simulink library "casper_library"  (Simulink 6.2)
PostLoadFcn:
  | % Stub definitions for mask variables
  | delay_depth=16;
  | n_bits=8;
  | bin_pt=7;
values from neighbouring files (symbols this model uses):
  add_latency = get_var('add_latency', 'defaults', defaults, varargin{:})    [biplex_core_init.m]    (also in butterfly_direct_init.m; dec_fir_init.m = get_var('add_latency','defaults', defaults, varargin{:}); fft_biplex_real_4x_init.m; fft_direct_init.m)
  BitWidth = get_var('BitWidth', 'defaults', defaults, varargin{:})    [biplex_core_init.m]    (also in butterfly_direct_init.m; fft_biplex_init.m; fft_biplex_real_2x_init.m; fft_biplex_real_4x_init.m)
  blockCountBits = ceil(log2(numBlocks))    [address_gen_vacc_v2_mask.m]
  blockRowBits = 0    [address_gen_vacc_v2_mask.m]
  mult_latency = get_var('mult_latency', 'defaults', defaults, varargin{:})    [biplex_core_init.m]    (also in butterfly_direct_init.m; dec_fir_init.m = get_var('mult_latency','defaults', defaults, varargin{:}); fft_biplex_real_4x_init.m; fft_direct_init.m)
  n_inputs = get_var('n_inputs', 'defaults', defaults, varargin{:})    [adder_tree_init.m]    (also in barrel_switcher_init.m; dec_fir_init.m = get_var('n_inputs','defaults', defaults, varargin{:}); fft_init.m; fft_unscrambler_init.m)
undefined symbols (not defined in the file or in its folder): acc_len, ant_bits, bit_growth, bit_rev, BitWidthIn, cmult_4bit_br, cmult_4bit_em, cmult_4bit_sl, CoeffBitWidth, DelayLen, n_ants, n_bits_out, pfb_coeff_gen_calc, PFBSize
libraries: xbsIndex_r3 x2630, casper_library x215, xps_library x24, fft_library x4
(part 5 of 21)

== system casper_library/Misc/adder_tree ==
  sync : Inport  Port=1  LatchInput=off
  din1 : Inport  Port=2  LatchInput=off
  din2 : Inport  Port=3  LatchInput=off
  addr1 : xbsIndex_r3/AddSub  mode=Addition  precision=Full  arith_type=Unsigned  n_bits=8  bin_pt=2  quantization=Truncate  overflow=Wrap  latency=1  explicit_period=off  period=1  use_carryin=off  use_carryout=off  en=off  dbl_ovrd=off  show_param=off  use_core=on  pipeline=on  use_rpm=on  gen_core=off
      settings: xl_area=[0, 0, 0, 0, 0, 0, 0]
  sync_delay : xbsIndex_r3/Delay  latency=1  reg_retiming=off  explicit_period=off  period=1  en=off  accept_only_valid=off  init_zero=on  dbl_ovrd=off  show_param=off
      settings: xl_area=[0, 0, 0, 0, 0, 0, 0]
  sync_out : Outport
  dout : Outport  Port=2
  wires:
  sync/1 -> sync_delay/1
  sync_delay/1 -> sync_out/1
  din1/1 -> addr1/1
  din2/1 -> addr1/2
  addr1/1 -> dout/1

== system casper_library/Misc/bit_reverse ==
  in : Inport  Port=1  LatchInput=off
  out : Outport
  wires:
  in/1 -> out/1

== system casper_library/Misc/c_to_ri ==
  c : Inport  Port=1  LatchInput=off
  force_im : xbsIndex_r3/Reinterpret  force_arith_type=on  arith_type="Signed  (2's comp)"  force_bin_pt=on  bin_pt=bin_pt  force_valid=on
  force_re : xbsIndex_r3/Reinterpret  force_arith_type=on  arith_type="Signed  (2's comp)"  force_bin_pt=on  bin_pt=bin_pt  force_valid=on
  slice_im : xbsIndex_r3/Slice  mode=Lower Bit Location + Width  nbits=n_bits  bit1=0  base1=MSB of Input  bit0=0  base0=LSB of Input  boolean_output=off  explicit_period=off  period=1  dbl_ovrd=off
  slice_re : xbsIndex_r3/Slice  mode=Upper Bit Location + Width  nbits=n_bits  bit1=0  base1=MSB of Input  bit0=0  base0=LSB of Input  boolean_output=off  explicit_period=off  period=1  dbl_ovrd=off
  re : Outport
  im : Outport  Port=2
  wires:
  slice_re/1 -> force_re/1
  slice_im/1 -> force_im/1
  force_re/1 -> re/1
  force_im/1 -> im/1
  c/1 -> slice_re/1, slice_im/1

== system casper_library/Misc/complex_addsub ==
  a : Inport  Port=1  LatchInput=off
  b : Inport  Port=2  LatchInput=off
  AddSub : xbsIndex_r3/AddSub  mode=Addition  precision=Full  arith_type=Unsigned  n_bits=8  bin_pt=2  quantization=Truncate  overflow=Wrap  latency=add_latency  explicit_period=off  period=1  use_carryin=off  use_carryout=off  en=off  dbl_ovrd=off  show_param=off  use_core=on  pipeline=off  use_rpm=on  gen_core=off
      settings: xl_area=[0, 0, 0, 0, 0, 0, 0]
  AddSub1 : xbsIndex_r3/AddSub  mode=Subtraction  precision=Full  arith_type=Unsigned  n_bits=8  bin_pt=2  quantization=Truncate  overflow=Wrap  latency=add_latency  explicit_period=off  period=1  use_carryin=off  use_carryout=off  en=off  dbl_ovrd=off  show_param=off  use_core=on  pipeline=off  use_rpm=on  gen_core=off
      settings: xl_area=[0, 0, 0, 0, 0, 0, 0]
  AddSub2 : xbsIndex_r3/AddSub  mode=Subtraction  precision=Full  arith_type=Unsigned  n_bits=8  bin_pt=2  quantization=Truncate  overflow=Wrap  latency=add_latency  explicit_period=off  period=1  use_carryin=off  use_carryout=off  en=off  dbl_ovrd=off  show_param=off  use_core=on  pipeline=off  use_rpm=on  gen_core=off
      settings: xl_area=[0, 0, 0, 0, 0, 0, 0]
  AddSub3 : xbsIndex_r3/AddSub  mode=Addition  precision=Full  arith_type=Unsigned  n_bits=8  bin_pt=2  quantization=Truncate  overflow=Wrap  latency=add_latency  explicit_period=off  period=1  use_carryin=off  use_carryout=off  en=off  dbl_ovrd=off  show_param=off  use_core=on  pipeline=off  use_rpm=on  gen_core=off
      settings: xl_area=[0, 0, 0, 0, 0, 0, 0]
  Convert{,1..3} (4 alike) : xbsIndex_r3/Convert  arith_type="Signed  (2's comp)"  n_bits=BitWidth  bin_pt=BitWidth - 1  quantization="Round  (unbiased: Even Values)"  overflow=Wrap  latency=add_latency  explicit_period=off  period=1  dbl_ovrd=off  show_param=off  inserted_by_tool=off  pipeline=off
      settings: xl_area=[0, 0, 0, 0, 0, 0, 0]
  Shift{,1..3} (4 alike) : xbsIndex_r3/Shift  shift_dir=Right  shift_bits=1  precision=Full  arith_type="Signed  (2's comp)"  n_bits=8  bin_pt=2  quantization=Truncate  overflow=Wrap  latency=0  explicit_period=off  period=1  en=off  dbl_ovrd=off  show_param=off
      settings: xl_area=[0, 0, 0, 0, 0, 0, 0]
  c_to_ri : casper_library/Misc/c_to_ri  n_bits=BitWidth  bin_pt=BitWidth-1
      settings: AttributesFormatString=18_17 r/i
  c_to_ri1 : casper_library/Misc/c_to_ri  n_bits=BitWidth  bin_pt=BitWidth-1
      settings: AttributesFormatString=18_17 r/i
  ri_to_c : casper_library/Misc/ri_to_c
  ri_to_c1 : casper_library/Misc/ri_to_c
  a+b : Outport
  a-b : Outport  Port=2
  wires:
  Shift3/1 -> Convert3/1
  Shift2/1 -> Convert2/1
  Shift1/1 -> Convert1/1
  Shift/1 -> Convert/1
  b/1 -> c_to_ri1/1
  ri_to_c1/1 -> a-b/1
  ri_to_c/1 -> a+b/1
  a/1 -> c_to_ri/1
  Convert2/1 -> ri_to_c/2
  Convert/1 -> ri_to_c/1
  c_to_ri1/2 -> AddSub3/2, AddSub2/2
  c_to_ri1/1 -> AddSub/2, AddSub1/1
  c_to_ri/2 -> AddSub3/1, AddSub2/1
  c_to_ri/1 -> AddSub/1, AddSub1/2
  AddSub3/1 -> Shift3/1
  AddSub2/1 -> Shift2/1
  AddSub1/1 -> Shift1/1
  AddSub/1 -> Shift/1
  Convert1/1 -> ri_to_c1/2
  Convert3/1 -> ri_to_c1/1

== system casper_library/Misc/cram ==
  In1 : Inport  Port=1  LatchInput=off
  In2 : Inport  Port=2  LatchInput=off
  In3 : Inport  Port=3  LatchInput=off
  In4 : Inport  Port=4  LatchInput=off
  Concat : S-Function  AncestorBlock=xbsIndex_r3/Concat  FunctionName=xlconcat  Parameters=sfcn_mwsv__  mask(Xilinx Bus Concatenator){num_inputs=4, explicit_period=off, period=1, dbl_ovrd=off}
      mask prompts: num_inputs "Number of Inputs"; explicit_period "Use Explicit Sample Period"; period "Sample Period  (use -1 to inherit first known input period)"; dbl_ovrd "Override with Doubles"
      mask help: Concatenates two or more inputs. Inputs must be unsigned with binary point at zero.
      mask init:
      | [designRoot, family, part, speed, package, simulinkPeriod, sysclkPeriod, dbl_ovrd, trimVbit] = xlSysgenSettings(gcb,1,1);
      | [bg,fg] = xlcmap('XBlock',dbl_ovrd);
      | iPos = get_param(gcb,'Position');
      | iWidth=iPos(3)-iPos(1); iHeight=iPos(4)-iPos(2);
      | iCx=iWidth/2;
      | iCy=iHeight/2;
      | [logoX, logoY] = xlogo(iPos);
      | 
      | 
      | 
      | 
      | % one time added for param list
      | numInputs = num_inputs + 1;
      | precision0 = 1;
      | latency = 0;
      | dblOvrd = dbl_ovrd;
      | explicitClk = explicit_period;
      | 
      | 
      | % just pass everything to s-function
      | sfcn_mwsv__ = get_param(gcb, 'MaskWSVariables');
      mask Help: eval('xlWeb(xlhtmldoclink(''Concat''))');
      mask StyleString: popup(2|3|4|5|6|7|8|9|10|11|12|13|14|15|16),checkbox,edit,checkbox
      mask CallbackString: |xlMagicCallback||
      mask Display:
      | patch([0 iWidth iWidth 0],[0 0 iHeight iHeight] , bg);
      | patch(logoX,logoY, fg);
      | port_label('input',1,'hi');
      | port_label('input',num_inputs+1,'lo');
      | port_label('output',1,'cat');
      | ;plot([0 0 iWidth iWidth 0], [0 iHeight iHeight 0 0]);
  Reinterp{1..4} (4 alike) : xbsIndex_r3/Reinterpret  force_arith_type=on  arith_type=Unsigned  force_bin_pt=on  bin_pt=0  force_valid=on
  Out : Outport
  wires:
  Concat/1 -> Out/1
  In1/1 -> Reinterp1/1
  Reinterp1/1 -> Concat/1
  In2/1 -> Reinterp2/1
  Reinterp2/1 -> Concat/2
  In3/1 -> Reinterp3/1
  Reinterp3/1 -> Concat/3
  In4/1 -> Reinterp4/1
  Reinterp4/1 -> Concat/4

== system casper_library/Misc/edge ==
  in : Inport  Port=1  LatchInput=off
  Delay4 : xbsIndex_r3/Delay  latency=1  reg_retiming=off  explicit_period=off  period=1  en=off  accept_only_valid=off  init_zero=on  dbl_ovrd=off  show_param=off
      settings: xl_area=[0, 0, 0, 0, 0, 0, 0]
  Logical3 : xbsIndex_r3/Logical  logical_function=XOR  inputs=2  precision=Full  arith_type=Unsigned  n_bits=8  bin_pt=2  align_bp=on  latency=0  explicit_period=off  period=1  en=off  dbl_ovrd=off  show_param=off
      settings: xl_area=[0, 0, 0, 0, 0, 0, 0]
  out : Outport
  wires:
  Logical3/1 -> out/1
  Delay4/1 -> Logical3/1
  in/1 -> Delay4/1, Logical3/2

== system casper_library/Misc/freeze_cntr ==
  en : Inport  Port=1  LatchInput=off
  rst : Inport  Port=2  LatchInput=off
  Counter3 : xbsIndex_r3/Counter  cnt_type=Free Running  n_bits=CounterBits + 1  bin_pt=0  arith_type=Unsigned  start_count=0  cnt_to=1023  cnt_by_val=1  operation=Up  explicit_period=on  period=1  load_pin=off  rst=on  en=on  dbl_ovrd=off  show_param=off  use_rpm=on  gen_core=off
      settings: xl_area=[0, 0, 0, 0, 0, 0, 0]
  Inverter : xbsIndex_r3/Inverter  latency=0  explicit_period=off  period=1  en=off  dbl_ovrd=off  show_param=off
      settings: xl_area=[0, 0, 0, 0, 0, 0, 0]
  Inverter1 : xbsIndex_r3/Inverter  latency=0  explicit_period=off  period=1  en=off  dbl_ovrd=off  show_param=off
      settings: xl_area=[0, 0, 0, 0, 0, 0, 0]
  Logical1 : xbsIndex_r3/Logical  logical_function=AND  inputs=2  precision=Full  arith_type=Unsigned  n_bits=8  bin_pt=2  align_bp=on  latency=0  explicit_period=off  period=1  en=off  dbl_ovrd=off  show_param=off
      settings: xl_area=[0, 0, 0, 0, 0, 0, 0]
  Logical5 : xbsIndex_r3/Logical  logical_function=AND  inputs=2  precision=Full  arith_type=Unsigned  n_bits=8  bin_pt=2  align_bp=on  latency=0  explicit_period=off  period=1  en=off  dbl_ovrd=off  show_param=off
      settings: xl_area=[0, 0, 0, 0, 0, 0, 0]
  enable : xbsIndex_r3/Slice  mode=Lower Bit Location + Width  nbits=CounterBits  bit1=0  base1=LSB of Input  bit0=0  base0=LSB of Input  boolean_output=off  explicit_period=off  period=1  dbl_ovrd=off
  enable1 : xbsIndex_r3/Slice  mode=Upper Bit Location + Width  nbits=1  bit1=0  base1=MSB of Input  bit0=0  base0=LSB of Input  boolean_output=on  explicit_period=off  period=1  dbl_ovrd=off
  addr : Outport
  we : Outport  Port=2
  done : Outport  Port=3
  wires:
  Logical1/1 -> we/1
  Inverter/1 -> Logical1/1
  Counter3/1 -> enable1/1, enable/1
  enable1/1 -> Inverter1/1, done/1
  en/1 -> Logical5/1
  Logical5/1 -> Logical1/2, Counter3/2
  rst/1 -> Inverter/1, Counter3/1
  enable/1 -> addr/1
  Inverter1/1 -> Logical5/2

== system casper_library/Misc/negedge ==
  In : Inport  Port=1  LatchInput=off
  Delay : xbsIndex_r3/Delay  latency=1  reg_retiming=off  explicit_period=off  period=1  en=off  accept_only_valid=off  init_zero=on  dbl_ovrd=off  show_param=off
      settings: xl_area=[0, 0, 0, 0, 0, 0, 0]
  Inverter : xbsIndex_r3/Inverter  latency=0  explicit_period=off  period=1  en=off  dbl_ovrd=off  show_param=off
      settings: xl_area=[0, 0, 0, 0, 0, 0, 0]
  Logical : xbsIndex_r3/Logical  logical_function=AND  inputs=2  precision=Full  arith_type=Unsigned  n_bits=8  bin_pt=2  align_bp=on  latency=0  explicit_period=off  period=1  en=off  dbl_ovrd=off  show_param=off
      settings: xl_area=[0, 0, 0, 0, 0, 0, 0]
  Out : Outport
  wires:
  Delay/1 -> Logical/1
  In/1 -> Delay/1, Inverter/1
  Logical/1 -> Out/1
  Inverter/1 -> Logical/2

== system casper_library/Misc/posedge ==
  In : Inport  Port=1  LatchInput=off
  Delay : xbsIndex_r3/Delay  latency=1  reg_retiming=off  explicit_period=off  period=1  en=off  accept_only_valid=off  init_zero=on  dbl_ovrd=off  show_param=off
      settings: xl_area=[0, 0, 0, 0, 0, 0, 0]
  Inverter : xbsIndex_r3/Inverter  latency=0  explicit_period=off  period=1  en=off  dbl_ovrd=off  show_param=off
      settings: xl_area=[0, 0, 0, 0, 0, 0, 0]
  Logical : xbsIndex_r3/Logical  logical_function=AND  inputs=2  precision=Full  arith_type=Unsigned  n_bits=8  bin_pt=2  align_bp=on  latency=0  explicit_period=off  period=1  en=off  dbl_ovrd=off  show_param=off
      settings: xl_area=[0, 0, 0, 0, 0, 0, 0]
  Out : Outport
  wires:
  Logical/1 -> Out/1
  In/1 -> Logical/2, Delay/1
  Inverter/1 -> Logical/1
  Delay/1 -> Inverter/1

== system casper_library/Misc/power ==
  c : Inport  Port=1  LatchInput=off
  c_to_ri : casper_library/Misc/c_to_ri  n_bits=BitWidth  bin_pt=BitWidth-1
      settings: AttributesFormatString=18_17 r/i
  imag_square : xbsIndex_r3/Mult  precision=Full  arith_type="Signed  (2's comp)"  n_bits=8  bin_pt=2  quantization=Truncate  overflow=Wrap  latency=3  explicit_period=off  period=1  en=off  dbl_ovrd=off  show_param=on  mult_type=Parallel  oversample=2  use_embedded=on  pipeline=on  use_rpm=on  placement_style=Rectangular Shape  gen_core=off
      settings: xl_area=[0, 0, 0, 0, 0, 0, 0]
  power_adder : xbsIndex_r3/AddSub  mode=Addition  precision=User Defined  arith_type=Unsigned  n_bits=BitWidth * 2  bin_pt=BitWidth * 2 - 1  quantization=Truncate  overflow=Wrap  latency=2  explicit_period=off  period=1  use_carryin=off  use_carryout=off  en=off  dbl_ovrd=off  show_param=off  use_core=on  pipeline=off  use_rpm=on  gen_core=off
      settings: xl_area=[0, 0, 0, 0, 0, 0, 0]
  real_square : xbsIndex_r3/Mult  precision=Full  arith_type="Signed  (2's comp)"  n_bits=8  bin_pt=2  quantization=Truncate  overflow=Wrap  latency=3  explicit_period=off  period=1  en=off  dbl_ovrd=off  show_param=on  mult_type=Parallel  oversample=2  use_embedded=on  pipeline=on  use_rpm=on  placement_style=Rectangular Shape  gen_core=off
      settings: xl_area=[0, 0, 0, 0, 0, 0, 0]
  power : Outport
  wires:
  c_to_ri/2 -> imag_square/1, imag_square/2
  c_to_ri/1 -> real_square/2, real_square/1
  c/1 -> c_to_ri/1
  real_square/1 -> power_adder/1
  imag_square/1 -> power_adder/2
  power_adder/1 -> power/1

== system casper_library/Misc/pulse_ext ==
  in : Inport  Port=1  LatchInput=off
  Constant5 : xbsIndex_r3/Constant  const=pulse_len  equ=P=C  arith_type=Unsigned  n_bits=bits  bin_pt=0  opselect=C  inp2=PCIN>>17  opr=+  inp1=P  carry=CIN  iostate=0  explicit_period=off  period=1  dbl_ovrd=off
  Counter3 : xbsIndex_r3/Counter  cnt_type=Free Running  n_bits=bits  bin_pt=0  arith_type=Unsigned  start_count=0  cnt_to=1023  cnt_by_val=1  operation=Up  explicit_period=on  period=1  load_pin=off  rst=on  en=on  dbl_ovrd=off  show_param=off  use_rpm=on  gen_core=off
      settings: xl_area=[0, 0, 0, 0, 0, 0, 0]
  Relational5 : xbsIndex_r3/Relational  mode=a!=b  latency=0  explicit_period=off  period=1  en=off  dbl_ovrd=off  show_param=off
      settings: xl_area=[0, 0, 0, 0, 0, 0, 0]
  posedge : Subsystem  Tag=Rising Edge Detector
  out : Outport
  wires:
  Counter3/1 -> Relational5/1
  Constant5/1 -> Relational5/2
  Relational5/1 -> Counter3/2, out/1
  in/1 -> posedge/1(In)
  posedge/1(Out) -> Counter3/1

== system casper_library/Misc/ri_to_c ==
  re : Inport  Port=1  LatchInput=off
  im : Inport  Port=2  LatchInput=off
  concat : xbsIndex_r3/Concat  num_inputs=2  explicit_period=off  period=1  dbl_ovrd=off
  force_im : xbsIndex_r3/Reinterpret  force_arith_type=on  arith_type=Unsigned  force_bin_pt=on  bin_pt=0  force_valid=on
  force_re : xbsIndex_r3/Reinterpret  force_arith_type=on  arith_type=Unsigned  force_bin_pt=on  bin_pt=0  force_valid=on
  c : Outport
  wires:
  force_re/1 -> concat/1
  force_im/1 -> concat/2
  re/1 -> force_re/1
  concat/1 -> c/1
  im/1 -> force_im/1

== system casper_library/Misc/stopwatch ==
  start : Inport  Port=1  LatchInput=off
  stop : Inport  Port=2  LatchInput=off
  reset : Inport  Port=3  LatchInput=off
  Constant1 : xbsIndex_r3/Constant  const=1  equ=P=C  arith_type=Boolean  n_bits=1  bin_pt=0  opselect=C  inp2=PCIN>>17  opr=+  inp1=P  carry=CIN  iostate=0  explicit_period=on  period=1  dbl_ovrd=off
  Constant8 : xbsIndex_r3/Constant  const=1  equ=P=C  arith_type=Boolean  n_bits=1  bin_pt=0  opselect=C  inp2=PCIN>>17  opr=+  inp1=P  carry=CIN  iostate=0  explicit_period=on  period=1  dbl_ovrd=off
  Counter1 : xbsIndex_r3/Counter  cnt_type=Free Running  n_bits=32  bin_pt=0  arith_type=Unsigned  start_count=0  cnt_to=Inf  cnt_by_val=1  operation=Up  explicit_period=off  period=1  load_pin=off  rst=on  en=on  dbl_ovrd=off  show_param=off  use_rpm=on  gen_core=off
      settings: xl_area=[0, 0, 0, 0, 0, 0, 0]
  Logical : xbsIndex_r3/Logical  logical_function=AND  inputs=2  precision=Full  arith_type=Unsigned  n_bits=8  bin_pt=2  align_bp=on  latency=0  explicit_period=off  period=1  en=off  dbl_ovrd=off  show_param=off
      settings: xl_area=[0, 0, 0, 0, 0, 0, 0]
  Logical1 : xbsIndex_r3/Logical  logical_function=OR  inputs=2  precision=Full  arith_type=Unsigned  n_bits=8  bin_pt=2  align_bp=on  latency=0  explicit_period=off  period=1  en=off  dbl_ovrd=off  show_param=off
      settings: xl_area=[0, 0, 0, 0, 0, 0, 0]
  Register1 : xbsIndex_r3/Register  init=0  reg_only_valid=off  explicit_period=off  period=1  rst=on  en=on  out_en=off  dbl_ovrd=off  show_param=off
      settings: xl_area=[0, 0, 0, 0, 0, 0, 0]
  Register3 : xbsIndex_r3/Register  init=0  reg_only_valid=off  explicit_period=off  period=1  rst=on  en=on  out_en=off  dbl_ovrd=off  show_param=off
      settings: xl_area=[0, 0, 0, 0, 0, 0, 0]
  count_out : Outport
  wires:
  Logical1/1 -> Register3/3
  stop/1 -> Register3/2
  Register1/1 -> Logical/2
  Register3/1 -> Logical/1
  Logical/1 -> Counter1/2
  reset/1 -> Logical1/2, Register1/2, Counter1/1
  start/1 -> Logical1/1, Register1/3
  Constant1/1 -> Register1/1
  Counter1/1 -> count_out/1
  Constant8/1 -> Register3/1

== system casper_library/Misc/uncram ==
  In : Inport  Port=1  LatchInput=off
  Reinterp1 : xbsIndex_r3/Reinterpret  force_arith_type=on  arith_type="Signed  (2's comp)"  force_bin_pt=on  bin_pt=17  force_valid=on
  Reinterp2 : xbsIndex_r3/Reinterpret  force_arith_type=on  arith_type="Signed  (2's comp)"  force_bin_pt=on  bin_pt=17  force_valid=on
  Slice1 : xbsIndex_r3/Slice  mode=Upper Bit Location + Width  nbits=18  bit1=0  base1=MSB of Input  bit0=0  base0=LSB of Input  boolean_output=off  explicit_period=off  period=1  dbl_ovrd=off
  Slice2 : xbsIndex_r3/Slice  mode=Upper Bit Location + Width  nbits=18  bit1=-18  base1=MSB of Input  bit0=0  base0=LSB of Input  boolean_output=off  explicit_period=off  period=1  dbl_ovrd=off
  Out1 : Outport
  Out2 : Outport  Port=2
  wires:
  Reinterp2/1 -> Out2/1
  Slice2/1 -> Reinterp2/1
  Reinterp1/1 -> Out1/1
  Slice1/1 -> Reinterp1/1
  In/1 -> Slice2/1, Slice1/1

== system casper_library/Multipliers/cmult ==
  a : Inport  Port=1  LatchInput=off
  b : Inport  Port=2  LatchInput=off
  c : Inport  Port=3  LatchInput=off
  d : Inport  Port=4  LatchInput=off
  cmult_4bit_br : casper_library/Multipliers/cmult_4bit_br  mult_latency=1  add_latency=0
  real : Outport
  imag : Outport  Port=2
  wires:
  a/1 -> cmult_4bit_br/1
  b/1 -> cmult_4bit_br/2
  c/1 -> cmult_4bit_br/3
  d/1 -> cmult_4bit_br/4
  cmult_4bit_br/1 -> real/1
  cmult_4bit_br/2 -> imag/1

== system casper_library/Multipliers/cmult* ==
  a : Inport  Port=1  LatchInput=off
  b : Inport  Port=2  LatchInput=off
  c : Inport  Port=3  LatchInput=off
  d : Inport  Port=4  LatchInput=off
  cmult_4bit_br* : casper_library/Multipliers/cmult_4bit_br*  mult_latency=1  add_latency=0
  real : Outport
  imag : Outport  Port=2
  wires:
  a/1 -> cmult_4bit_br*/1
  b/1 -> cmult_4bit_br*/2
  c/1 -> cmult_4bit_br*/3
  d/1 -> cmult_4bit_br*/4
  cmult_4bit_br*/1 -> real/1
  cmult_4bit_br*/2 -> imag/1

== system casper_library/Multipliers/cmult_4bit_br ==
  a : Inport  Port=1  LatchInput=off
  b : Inport  Port=2  LatchInput=off
  c : Inport  Port=3  LatchInput=off
  d : Inport  Port=4  LatchInput=off
  Concat{,1..3} (4 alike) : xbsIndex_r3/Concat  num_inputs=2  explicit_period=off  period=1  dbl_ovrd=off
  ROM : xbsIndex_r3/ROM  depth=256  initVector=transpose(transpose([0:7 -8:-1]) * [0:7 -8:-1]) / 64  arith_type="Signed  (2's comp)"  n_bits=8  bin_pt=6  latency=mult_latency  init_zero=on  explicit_period=off  period=1  rst=off  init_reg=0  en=off  dbl_ovrd=off  show_param=off  distributed_mem=off  use_rpm=off  gen_core=off
      settings: xl_area=[0 0 1 0 0 0 0]
  ROM1 : xbsIndex_r3/ROM  depth=256  initVector=transpose([0:7 -8:-1]) * [0:7 -8:-1] / 64  arith_type="Signed  (2's comp)"  n_bits=8  bin_pt=6  latency=mult_latency  init_zero=on  explicit_period=off  period=1  rst=off  init_reg=0  en=off  dbl_ovrd=off  show_param=off  distributed_mem=off  use_rpm=off  gen_core=off
      settings: xl_area=[0 0 1 0 0 0 0]
  ROM2 : xbsIndex_r3/ROM  depth=256  initVector=transpose([0:7 -8:-1]) * [0:7 -8:-1] / 64  arith_type="Signed  (2's comp)"  n_bits=8  bin_pt=6  latency=mult_latency  init_zero=on  explicit_period=off  period=1  rst=off  init_reg=0  en=off  dbl_ovrd=off  show_param=off  distributed_mem=off  use_rpm=off  gen_core=off
      settings: xl_area=[0 0 1 0 0 0 0]
  ROM3 : xbsIndex_r3/ROM  depth=256  initVector=transpose([0:7 -8:-1]) * [0:7 -8:-1] / 64  arith_type="Signed  (2's comp)"  n_bits=8  bin_pt=6  latency=mult_latency  init_zero=on  explicit_period=off  period=1  rst=off  init_reg=0  en=off  dbl_ovrd=off  show_param=off  distributed_mem=off  use_rpm=off  gen_core=off
      settings: xl_area=[0 0 1 0 0 0 0]
  Reinterpret{1..8} (8 alike) : xbsIndex_r3/Reinterpret  force_arith_type=on  arith_type=Unsigned  force_bin_pt=on  bin_pt=0  force_valid=on
  Resource Estimator : xbsIndex_r3/Resource Estimator  Tag=resEstTag  xl_estimator_area=[10 18 4 16 0 0 0]  xl_use_estimator_area=off  simulink_period=1  mrp_directory=B:\projects\eor_eight_station
      settings: AttributesFormatString=Resource\nEstimator
  imag_sum : xbsIndex_r3/AddSub  mode=Addition  precision=Full  arith_type=Unsigned  n_bits=8  bin_pt=2  quantization=Truncate  overflow=Wrap  latency=add_latency  explicit_period=off  period=1  use_carryin=off  use_carryout=off  en=off  dbl_ovrd=off  show_param=off  use_core=on  pipeline=off  use_rpm=on  gen_core=off
      settings: xl_area=[5 9 0 8 0 0 0]
  real_sum : xbsIndex_r3/AddSub  mode=Subtraction  precision=Full  arith_type=Unsigned  n_bits=8  bin_pt=2  quantization=Truncate  overflow=Wrap  latency=add_latency  explicit_period=off  period=1  use_carryin=off  use_carryout=off  en=off  dbl_ovrd=off  show_param=off  use_core=on  pipeline=off  use_rpm=on  gen_core=off
      settings: xl_area=[5 9 0 8 0 0 0]
  real : Outport
  imag : Outport  Port=2
  wires:
  ROM/1 -> real_sum/1
  ROM1/1 -> real_sum/2
  ROM2/1 -> imag_sum/1
  ROM3/1 -> imag_sum/2
  a/1 -> Reinterpret3/1, Reinterpret7/1
  c/1 -> Reinterpret1/1, Reinterpret6/1
  b/1 -> Reinterpret2/1, Reinterpret5/1
  d/1 -> Reinterpret4/1, Reinterpret8/1
  real_sum/1 -> real/1
  imag_sum/1 -> imag/1
  Concat/1 -> ROM/1
  Concat1/1 -> ROM1/1
  Concat2/1 -> ROM2/1
  Concat3/1 -> ROM3/1
  Reinterpret3/1 -> Concat/1
  Reinterpret1/1 -> Concat/2
  Reinterpret2/1 -> Concat1/1
  Reinterpret4/1 -> Concat1/2
  Reinterpret5/1 -> Concat2/1
  Reinterpret6/1 -> Concat2/2
  Reinterpret7/1 -> Concat3/1
  Reinterpret8/1 -> Concat3/2

== system casper_library/Multipliers/cmult_4bit_br* ==
  a : Inport  Port=1  LatchInput=off
  b : Inport  Port=2  LatchInput=off
  c : Inport  Port=3  LatchInput=off
  d : Inport  Port=4  LatchInput=off
  Concat{,1..3} (4 alike) : xbsIndex_r3/Concat  num_inputs=2  explicit_period=off  period=1  dbl_ovrd=off
  ROM : xbsIndex_r3/ROM  depth=256  initVector=transpose(transpose([0:7 -8:-1]) * [0:7 -8:-1]) / 64  arith_type="Signed  (2's comp)"  n_bits=8  bin_pt=6  latency=mult_latency  init_zero=on  explicit_period=off  period=1  rst=off  init_reg=0  en=off  dbl_ovrd=off  show_param=off  distributed_mem=off  use_rpm=off  gen_core=off
      settings: xl_area=[0 0 1 0 0 0 0]
  ROM1 : xbsIndex_r3/ROM  depth=256  initVector=transpose([0:7 -8:-1]) * [0:7 -8:-1] / 64  arith_type="Signed  (2's comp)"  n_bits=8  bin_pt=6  latency=mult_latency  init_zero=on  explicit_period=off  period=1  rst=off  init_reg=0  en=off  dbl_ovrd=off  show_param=off  distributed_mem=off  use_rpm=off  gen_core=off
      settings: xl_area=[0 0 1 0 0 0 0]
  ROM2 : xbsIndex_r3/ROM  depth=256  initVector=transpose([0:7 -8:-1]) * [0:7 -8:-1] / 64  arith_type="Signed  (2's comp)"  n_bits=8  bin_pt=6  latency=mult_latency  init_zero=on  explicit_period=off  period=1  rst=off  init_reg=0  en=off  dbl_ovrd=off  show_param=off  distributed_mem=off  use_rpm=off  gen_core=off
      settings: xl_area=[0 0 1 0 0 0 0]
  ROM3 : xbsIndex_r3/ROM  depth=256  initVector=transpose([0:7 -8:-1]) * [0:7 -8:-1] / 64  arith_type="Signed  (2's comp)"  n_bits=8  bin_pt=6  latency=mult_latency  init_zero=on  explicit_period=off  period=1  rst=off  init_reg=0  en=off  dbl_ovrd=off  show_param=off  distributed_mem=off  use_rpm=off  gen_core=off
      settings: xl_area=[0 0 1 0 0 0 0]
  Reinterpret{1..8} (8 alike) : xbsIndex_r3/Reinterpret  force_arith_type=on  arith_type=Unsigned  force_bin_pt=on  bin_pt=0  force_valid=on
  Resource Estimator : xbsIndex_r3/Resource Estimator  Tag=resEstTag  xl_estimator_area=[10 18 4 16 0 0 0]  xl_use_estimator_area=off  simulink_period=1  mrp_directory=B:\projects\eor_eight_station
      settings: AttributesFormatString=Resource\nEstimator
  imag_sum : xbsIndex_r3/AddSub  mode=Subtraction  precision=Full  arith_type=Unsigned  n_bits=8  bin_pt=2  quantization=Truncate  overflow=Wrap  latency=add_latency  explicit_period=off  period=1  use_carryin=off  use_carryout=off  en=off  dbl_ovrd=off  show_param=off  use_core=on  pipeline=off  use_rpm=on  gen_core=off
      settings: xl_area=[5 9 0 8 0 0 0]
  real_sum : xbsIndex_r3/AddSub  mode=Addition  precision=Full  arith_type=Unsigned  n_bits=8  bin_pt=2  quantization=Truncate  overflow=Wrap  latency=add_latency  explicit_period=off  period=1  use_carryin=off  use_carryout=off  en=off  dbl_ovrd=off  show_param=off  use_core=on  pipeline=off  use_rpm=on  gen_core=off
      settings: xl_area=[5 9 0 8 0 0 0]
  real : Outport
  imag : Outport  Port=2
  wires:
  Reinterpret8/1 -> Concat3/2
  Reinterpret7/1 -> Concat3/1
  Reinterpret6/1 -> Concat2/2
  Reinterpret5/1 -> Concat2/1
  Reinterpret4/1 -> Concat1/2
  Reinterpret2/1 -> Concat1/1
  Reinterpret1/1 -> Concat/2
  Reinterpret3/1 -> Concat/1
  Concat3/1 -> ROM3/1
  Concat2/1 -> ROM2/1
  Concat1/1 -> ROM1/1
  Concat/1 -> ROM/1
  imag_sum/1 -> imag/1
  real_sum/1 -> real/1
  d/1 -> Reinterpret8/1, Reinterpret4/1
  b/1 -> Reinterpret5/1, Reinterpret2/1
  c/1 -> Reinterpret6/1, Reinterpret1/1
  a/1 -> Reinterpret7/1, Reinterpret3/1
  ROM3/1 -> imag_sum/2
  ROM2/1 -> imag_sum/1
  ROM1/1 -> real_sum/2
  ROM/1 -> real_sum/1

== system casper_library/Multipliers/cmult_4bit_em ==
  a : Inport  Port=1  LatchInput=off
  b : Inport  Port=2  LatchInput=off
  c : Inport  Port=3  LatchInput=off
  d : Inport  Port=4  LatchInput=off
  Resource Estimator : xbsIndex_r3/Resource Estimator  Tag=resEstTag  xl_estimator_area=[26 18 0 48 0 4 0]  xl_use_estimator_area=off  simulink_period=1  mrp_directory=B:\projects\eor_eight_station
      settings: AttributesFormatString=Resource\nEstimator
  ac : xbsIndex_r3/Mult  precision=Full  arith_type="Signed  (2's comp)"  n_bits=8  bin_pt=2  quantization=Truncate  overflow=Wrap  latency=mult_latency  explicit_period=off  period=1  en=off  dbl_ovrd=off  show_param=on  mult_type=Parallel  oversample=2  use_embedded=on  pipeline=on  use_rpm=on  placement_style=Rectangular Shape  gen_core=off
      settings: xl_area=[4 0 0 8 0 1 0]
  ad : xbsIndex_r3/Mult  precision=Full  arith_type="Signed  (2's comp)"  n_bits=8  bin_pt=2  quantization=Truncate  overflow=Wrap  latency=mult_latency  explicit_period=off  period=1  en=off  dbl_ovrd=off  show_param=on  mult_type=Parallel  oversample=2  use_embedded=on  pipeline=on  use_rpm=on  placement_style=Rectangular Shape  gen_core=off
      settings: xl_area=[4 0 0 8 0 1 0]
  bc : xbsIndex_r3/Mult  precision=Full  arith_type="Signed  (2's comp)"  n_bits=8  bin_pt=2  quantization=Truncate  overflow=Wrap  latency=mult_latency  explicit_period=off  period=1  en=off  dbl_ovrd=off  show_param=on  mult_type=Parallel  oversample=2  use_embedded=on  pipeline=on  use_rpm=on  placement_style=Rectangular Shape  gen_core=off
      settings: xl_area=[4 0 0 8 0 1 0]
  bd : xbsIndex_r3/Mult  precision=Full  arith_type="Signed  (2's comp)"  n_bits=8  bin_pt=2  quantization=Truncate  overflow=Wrap  latency=mult_latency  explicit_period=off  period=1  en=off  dbl_ovrd=off  show_param=on  mult_type=Parallel  oversample=2  use_embedded=on  pipeline=on  use_rpm=on  placement_style=Rectangular Shape  gen_core=off
      settings: xl_area=[4 0 0 8 0 1 0]
  imag_sum : xbsIndex_r3/AddSub  mode=Addition  precision=Full  arith_type=Unsigned  n_bits=8  bin_pt=2  quantization=Truncate  overflow=Wrap  latency=add_latency  explicit_period=off  period=1  use_carryin=off  use_carryout=off  en=off  dbl_ovrd=off  show_param=off  use_core=on  pipeline=off  use_rpm=on  gen_core=off
      settings: xl_area=[5 9 0 8 0 0 0]
  real_sum : xbsIndex_r3/AddSub  mode=Subtraction  precision=Full  arith_type=Unsigned  n_bits=8  bin_pt=2  quantization=Truncate  overflow=Wrap  latency=add_latency  explicit_period=off  period=1  use_carryin=off  use_carryout=off  en=off  dbl_ovrd=off  show_param=off  use_core=on  pipeline=off  use_rpm=on  gen_core=off
      settings: xl_area=[5 9 0 8 0 0 0]
  real : Outport
  imag : Outport  Port=2
  wires:
  ac/1 -> real_sum/1
  bd/1 -> real_sum/2
  bc/1 -> imag_sum/1
  ad/1 -> imag_sum/2
  a/1 -> ad/1, ac/1
  c/1 -> bc/2, ac/2
  b/1 -> bc/1, bd/1
  d/1 -> ad/2, bd/2
  real_sum/1 -> real/1
  imag_sum/1 -> imag/1

== system casper_library/Multipliers/cmult_4bit_em* ==
  a : Inport  Port=1  LatchInput=off
  b : Inport  Port=2  LatchInput=off
  c : Inport  Port=3  LatchInput=off
  d : Inport  Port=4  LatchInput=off
  Resource Estimator : xbsIndex_r3/Resource Estimator  Tag=resEstTag  xl_estimator_area=[26 18 0 48 0 4 0]  xl_use_estimator_area=off  simulink_period=1  mrp_directory=B:\projects\eor_eight_station
      settings: AttributesFormatString=Resource\nEstimator
  ac : xbsIndex_r3/Mult  precision=Full  arith_type="Signed  (2's comp)"  n_bits=8  bin_pt=2  quantization=Truncate  overflow=Wrap  latency=mult_latency  explicit_period=off  period=1  en=off  dbl_ovrd=off  show_param=on  mult_type=Parallel  oversample=2  use_embedded=on  pipeline=on  use_rpm=on  placement_style=Rectangular Shape  gen_core=off
      settings: xl_area=[4 0 0 8 0 1 0]
  ad : xbsIndex_r3/Mult  precision=Full  arith_type="Signed  (2's comp)"  n_bits=8  bin_pt=2  quantization=Truncate  overflow=Wrap  latency=mult_latency  explicit_period=off  period=1  en=off  dbl_ovrd=off  show_param=on  mult_type=Parallel  oversample=2  use_embedded=on  pipeline=on  use_rpm=on  placement_style=Rectangular Shape  gen_core=off
      settings: xl_area=[4 0 0 8 0 1 0]
  bc : xbsIndex_r3/Mult  precision=Full  arith_type="Signed  (2's comp)"  n_bits=8  bin_pt=2  quantization=Truncate  overflow=Wrap  latency=mult_latency  explicit_period=off  period=1  en=off  dbl_ovrd=off  show_param=on  mult_type=Parallel  oversample=2  use_embedded=on  pipeline=on  use_rpm=on  placement_style=Rectangular Shape  gen_core=off
      settings: xl_area=[4 0 0 8 0 1 0]
  bd : xbsIndex_r3/Mult  precision=Full  arith_type="Signed  (2's comp)"  n_bits=8  bin_pt=2  quantization=Truncate  overflow=Wrap  latency=mult_latency  explicit_period=off  period=1  en=off  dbl_ovrd=off  show_param=on  mult_type=Parallel  oversample=2  use_embedded=on  pipeline=on  use_rpm=on  placement_style=Rectangular Shape  gen_core=off
      settings: xl_area=[4 0 0 8 0 1 0]
  imag_sum : xbsIndex_r3/AddSub  mode=Subtraction  precision=Full  arith_type=Unsigned  n_bits=8  bin_pt=2  quantization=Truncate  overflow=Wrap  latency=add_latency  explicit_period=off  period=1  use_carryin=off  use_carryout=off  en=off  dbl_ovrd=off  show_param=off  use_core=on  pipeline=off  use_rpm=on  gen_core=off
      settings: xl_area=[5 9 0 8 0 0 0]
  real_sum : xbsIndex_r3/AddSub  mode=Addition  precision=Full  arith_type=Unsigned  n_bits=8  bin_pt=2  quantization=Truncate  overflow=Wrap  latency=add_latency  explicit_period=off  period=1  use_carryin=off  use_carryout=off  en=off  dbl_ovrd=off  show_param=off  use_core=on  pipeline=off  use_rpm=on  gen_core=off
      settings: xl_area=[5 9 0 8 0 0 0]
  real : Outport
  imag : Outport  Port=2
  wires:
  imag_sum/1 -> imag/1
  real_sum/1 -> real/1
  d/1 -> bd/2, ad/2
  b/1 -> bd/1, bc/1
  c/1 -> ac/2, bc/2
  a/1 -> ac/1, ad/1
  ad/1 -> imag_sum/2
  bc/1 -> imag_sum/1
  bd/1 -> real_sum/2
  ac/1 -> real_sum/1

== system casper_library/Multipliers/cmult_4bit_sl ==
  a : Inport  Port=1  LatchInput=off
  b : Inport  Port=2  LatchInput=off
  c : Inport  Port=3  LatchInput=off
  d : Inport  Port=4  LatchInput=off
  ac : xbsIndex_r3/Mult  precision=Full  arith_type="Signed  (2's comp)"  n_bits=7  bin_pt=6  quantization=Truncate  overflow=Wrap  latency=mult_latency  explicit_period=off  period=1  en=off  dbl_ovrd=off  show_param=on  mult_type=Parallel  oversample=2  use_embedded=off  pipeline=off  use_rpm=on  placement_style=Rectangular Shape  gen_core=off
      settings: xl_area=[10 7 0 17 0 0 0]
  ad : xbsIndex_r3/Mult  precision=Full  arith_type="Signed  (2's comp)"  n_bits=7  bin_pt=6  quantization=Truncate  overflow=Wrap  latency=mult_latency  explicit_period=off  period=1  en=off  dbl_ovrd=off  show_param=on  mult_type=Parallel  oversample=2  use_embedded=off  pipeline=off  use_rpm=on  placement_style=Rectangular Shape  gen_core=off
      settings: xl_area=[10 7 0 17 0 0 0]
  bc : xbsIndex_r3/Mult  precision=Full  arith_type="Signed  (2's comp)"  n_bits=7  bin_pt=6  quantization=Truncate  overflow=Wrap  latency=mult_latency  explicit_period=off  period=1  en=off  dbl_ovrd=off  show_param=on  mult_type=Parallel  oversample=2  use_embedded=off  pipeline=off  use_rpm=on  placement_style=Rectangular Shape  gen_core=off
      settings: xl_area=[10 7 0 17 0 0 0]
  bd : xbsIndex_r3/Mult  precision=Full  arith_type="Signed  (2's comp)"  n_bits=7  bin_pt=6  quantization=Truncate  overflow=Wrap  latency=mult_latency  explicit_period=off  period=1  en=off  dbl_ovrd=off  show_param=on  mult_type=Parallel  oversample=2  use_embedded=off  pipeline=off  use_rpm=on  placement_style=Rectangular Shape  gen_core=off
      settings: xl_area=[10 7 0 17 0 0 0]
  imag_sum : xbsIndex_r3/AddSub  mode=Addition  precision=Full  arith_type=Unsigned  n_bits=8  bin_pt=2  quantization=Truncate  overflow=Wrap  latency=add_latency  explicit_period=off  period=1  use_carryin=off  use_carryout=off  en=off  dbl_ovrd=off  show_param=off  use_core=on  pipeline=off  use_rpm=on  gen_core=off
      settings: xl_area=[4 8 0 7 0 0 0]
  real_sum : xbsIndex_r3/AddSub  mode=Subtraction  precision=Full  arith_type=Unsigned  n_bits=8  bin_pt=2  quantization=Truncate  overflow=Wrap  latency=add_latency  explicit_period=off  period=1  use_carryin=off  use_carryout=off  en=off  dbl_ovrd=off  show_param=off  use_core=on  pipeline=off  use_rpm=on  gen_core=off
      settings: xl_area=[4 8 0 7 0 0 0]
  real : Outport
  imag : Outport  Port=2
  wires:
  imag_sum/1 -> imag/1
  real_sum/1 -> real/1
  d/1 -> bd/2, ad/2
  b/1 -> bd/1, bc/1
  c/1 -> ac/2, bc/2
  a/1 -> ac/1, ad/1
  ad/1 -> imag_sum/2
  bc/1 -> imag_sum/1
  bd/1 -> real_sum/2
  ac/1 -> real_sum/1

== system casper_library/Multipliers/cmult_4bit_sl* ==
  a : Inport  Port=1  LatchInput=off
  b : Inport  Port=2  LatchInput=off
  c : Inport  Port=3  LatchInput=off
  d : Inport  Port=4  LatchInput=off
  ac : xbsIndex_r3/Mult  precision=Full  arith_type="Signed  (2's comp)"  n_bits=7  bin_pt=6  quantization=Truncate  overflow=Wrap  latency=mult_latency  explicit_period=off  period=1  en=off  dbl_ovrd=off  show_param=on  mult_type=Parallel  oversample=2  use_embedded=off  pipeline=off  use_rpm=on  placement_style=Rectangular Shape  gen_core=off
      settings: xl_area=[10 7 0 17 0 0 0]
  ad : xbsIndex_r3/Mult  precision=Full  arith_type="Signed  (2's comp)"  n_bits=7  bin_pt=6  quantization=Truncate  overflow=Wrap  latency=mult_latency  explicit_period=off  period=1  en=off  dbl_ovrd=off  show_param=on  mult_type=Parallel  oversample=2  use_embedded=off  pipeline=off  use_rpm=on  placement_style=Rectangular Shape  gen_core=off
      settings: xl_area=[10 7 0 17 0 0 0]
  bc : xbsIndex_r3/Mult  precision=Full  arith_type="Signed  (2's comp)"  n_bits=7  bin_pt=6  quantization=Truncate  overflow=Wrap  latency=mult_latency  explicit_period=off  period=1  en=off  dbl_ovrd=off  show_param=on  mult_type=Parallel  oversample=2  use_embedded=off  pipeline=off  use_rpm=on  placement_style=Rectangular Shape  gen_core=off
      settings: xl_area=[10 7 0 17 0 0 0]
  bd : xbsIndex_r3/Mult  precision=Full  arith_type="Signed  (2's comp)"  n_bits=7  bin_pt=6  quantization=Truncate  overflow=Wrap  latency=mult_latency  explicit_period=off  period=1  en=off  dbl_ovrd=off  show_param=on  mult_type=Parallel  oversample=2  use_embedded=off  pipeline=off  use_rpm=on  placement_style=Rectangular Shape  gen_core=off
      settings: xl_area=[10 7 0 17 0 0 0]
  imag_sum : xbsIndex_r3/AddSub  mode=Subtraction  precision=Full  arith_type=Unsigned  n_bits=8  bin_pt=2  quantization=Truncate  overflow=Wrap  latency=add_latency  explicit_period=off  period=1  use_carryin=off  use_carryout=off  en=off  dbl_ovrd=off  show_param=off  use_core=on  pipeline=off  use_rpm=on  gen_core=off
      settings: xl_area=[4 8 0 7 0 0 0]
  real_sum : xbsIndex_r3/AddSub  mode=Addition  precision=Full  arith_type=Unsigned  n_bits=8  bin_pt=2  quantization=Truncate  overflow=Wrap  latency=add_latency  explicit_period=off  period=1  use_carryin=off  use_carryout=off  en=off  dbl_ovrd=off  show_param=off  use_core=on  pipeline=off  use_rpm=on  gen_core=off
      settings: xl_area=[4 8 0 7 0 0 0]
  real : Outport
  imag : Outport  Port=2
  wires:
  ac/1 -> real_sum/1
  bd/1 -> real_sum/2
  bc/1 -> imag_sum/1
  ad/1 -> imag_sum/2
  a/1 -> ad/1, ac/1
  c/1 -> bc/2, ac/2
  b/1 -> bc/1, bd/1
  d/1 -> ad/2, bd/2
  real_sum/1 -> real/1
  imag_sum/1 -> imag/1

== system casper_library/PFBs/first_tap ==
  din : Inport  Port=1  LatchInput=off
  sync : Inport  Port=2  LatchInput=off
  Mult : xbsIndex_r3/Mult  precision=Full  arith_type="Signed  (2's comp)"  n_bits=8  bin_pt=2  quantization=Truncate  overflow=Wrap  latency=mult_latency  explicit_period=off  period=1  en=off  dbl_ovrd=off  show_param=on  mult_type=Parallel  oversample=2  use_embedded=on  pipeline=on  use_rpm=on  placement_style=Rectangular Shape  gen_core=off
      settings: xl_area=[0, 0, 0, 0, 0, 0, 0]
  Mult1 : xbsIndex_r3/Mult  precision=Full  arith_type="Signed  (2's comp)"  n_bits=8  bin_pt=2  quantization=Truncate  overflow=Wrap  latency=mult_latency  explicit_period=off  period=1  en=off  dbl_ovrd=off  show_param=on  mult_type=Parallel  oversample=2  use_embedded=on  pipeline=on  use_rpm=on  placement_style=Rectangular Shape  gen_core=off
      settings: xl_area=[0, 0, 0, 0, 0, 0, 0]
  Reinterpret : xbsIndex_r3/Reinterpret  force_arith_type=on  arith_type="Signed  (2's comp)"  force_bin_pt=on  bin_pt=CoeffBitWidth - 1  force_valid=on
  Slice : xbsIndex_r3/Slice  mode=Lower Bit Location + Width  nbits=CoeffBitWidth  bit1=0  base1=MSB of Input  bit0=0  base0=LSB of Input  boolean_output=off  explicit_period=off  period=1  dbl_ovrd=off
  Slice1 : xbsIndex_r3/Slice  mode=Two Bit Locations  nbits=CoeffBitWidth * (TotalTaps - 1)  bit1=0  base1=MSB of Input  bit0=CoeffBitWidth  base0=LSB of Input  boolean_output=off  explicit_period=off  period=1  dbl_ovrd=off
  c_to_ri : casper_library/Misc/c_to_ri  n_bits=BitWidthIn  bin_pt=BitWidthIn-1
      settings: AttributesFormatString=8_7 r/i
  delay : Subsystem  BlockChoice=delay_bram
      link override delay_bram: DelayLen=2^(PFBSize-n_inputs)  bram_latency=bram_latency
      settings: AttributesFormatString=%<BlockChoice>  TemplateBlock=casper_library/Delays/delay  MemberBlocks=delay_bram,delay_slr
  pfb_coeff_gen : Subsystem  AncestorBlock=casper_library/PFBs/pfb_coeff_gen  mask(pfb_coeff_gen){PFBSize=11, CoeffBitWidth=8, TotalTaps=4, CoeffDistMem=1, WindowType=hamming, bram_latency=2, n_inputs=0, nput=0, fwidth=1}
      mask prompts: PFBSize "Size of PFB: (2^? pnts)"; CoeffBitWidth "Bitwidth of Coefficients:"; TotalTaps "Total Number of Taps:"; CoeffDistMem "Implement Coeff Gen in Distributed Memory"; WindowType "Windowing Function:"; bram_latency "BRAM Latency"; n_inputs "Number of Simultaneous Inputs: (2^?)"; nput "This is input number:"; fwidth "Bin Width (normal=1)"
      mask init: same as casper_library/PFBs/pfb_coeff_gen
      settings: AttributesFormatString=PFBSize=11, n_inputs=0, taps=4
  ri_to_c : Subsystem
  sync_delay : casper_library/Delays/sync_delay  DelayLen=2^(PFBSize-n_inputs)
  dout : Outport
  sync_out : Outport  Port=2
  coeff_out : Outport  Port=3
  taps_out : Outport  Port=4
  wires:
  ri_to_c/1(c) -> taps_out/1
  Mult/1 -> ri_to_c/2(im)
  Mult1/1 -> ri_to_c/1(re)
  c_to_ri/2 -> Mult/1
  c_to_ri/1 -> Mult1/1
  pfb_coeff_gen/3(coeff) -> Slice1/1, Slice/1
  pfb_coeff_gen/2(sync_out) -> sync_delay/1
  sync/1 -> pfb_coeff_gen/2(sync)
  pfb_coeff_gen/1(dout) -> delay/1(In1), c_to_ri/1
  din/1 -> pfb_coeff_gen/1(din)
  delay/1(Out1) -> dout/1
  sync_delay/1 -> sync_out/1
  Slice1/1 -> coeff_out/1
  Slice/1 -> Reinterpret/1
  Reinterpret/1 -> Mult1/2, Mult/2

== system casper_library/PFBs/first_tap_real ==
  din : Inport  Port=1  LatchInput=off
  sync : Inport  Port=2  LatchInput=off
  Mult : xbsIndex_r3/Mult  precision=Full  arith_type="Signed  (2's comp)"  n_bits=8  bin_pt=2  quantization=Truncate  overflow=Wrap  latency=mult_latency  explicit_period=off  period=1  en=off  dbl_ovrd=off  show_param=on  mult_type=Parallel  oversample=2  use_embedded=on  pipeline=on  use_rpm=on  placement_style=Rectangular Shape  gen_core=off
      settings: xl_area=[0, 0, 0, 0, 0, 0, 0]
  Reinterpret : xbsIndex_r3/Reinterpret  force_arith_type=on  arith_type="Signed  (2's comp)"  force_bin_pt=on  bin_pt=CoeffBitWidth - 1  force_valid=on
  Reinterpret1 : xbsIndex_r3/Reinterpret  force_arith_type=on  arith_type=Unsigned  force_bin_pt=on  bin_pt=0  force_valid=on
  Reinterpret2 : xbsIndex_r3/Reinterpret  force_arith_type=on  arith_type="Signed  (2's comp)"  force_bin_pt=on  bin_pt=BitWidthIn - 1  force_valid=on
  Slice : xbsIndex_r3/Slice  mode=Lower Bit Location + Width  nbits=CoeffBitWidth  bit1=0  base1=MSB of Input  bit0=0  base0=LSB of Input  boolean_output=off  explicit_period=off  period=1  dbl_ovrd=off
  Slice1 : xbsIndex_r3/Slice  mode=Two Bit Locations  nbits=CoeffBitWidth * (TotalTaps - 1)  bit1=0  base1=MSB of Input  bit0=CoeffBitWidth  base0=LSB of Input  boolean_output=off  explicit_period=off  period=1  dbl_ovrd=off
  delay : Subsystem  BlockChoice=delay_bram
      link override delay_bram: DelayLen=2^(PFBSize-n_inputs)  bram_latency=bram_latency
      link override delay_bram/Constant2: equ=P=C
      settings: AttributesFormatString=%<BlockChoice>  TemplateBlock=casper_library/Delays/delay  MemberBlocks=delay_bram,delay_slr
  pfb_coeff_gen : Subsystem  AncestorBlock=casper_library/PFBs/pfb_coeff_gen  mask(pfb_coeff_gen){PFBSize=8, CoeffBitWidth=8, TotalTaps=2, CoeffDistMem=1, CoeffRound=0, WindowType=hamming, bram_latency=2, n_inputs=2, nput=0, fwidth=1}
      mask prompts: PFBSize "Size of PFB: (2^? pnts)"; CoeffBitWidth "Bitwidth of Coefficients:"; TotalTaps "Total Number of Taps:"; CoeffDistMem "Implement Coeff Gen in Distributed Memory"; CoeffRound "Round-off Coefficients"; WindowType "Windowing Function:"; bram_latency "BRAM Latency"; n_inputs "Number of Simultaneous Inputs: (2^?)"; nput "This is input number:"; fwidth "Bin Width (normal=1)"
      mask init:
      | pfb_coeff_gen_init(gcb, ...
      |     'PFBSize', PFBSize, ...
      |     'CoeffBitWidth', CoeffBitWidth, ...
      |     'CoeffRound', CoeffRound, ...
      |     'TotalTaps', TotalTaps, ...
      |     'CoeffDistMem', CoeffDistMem, ...
      |     'WindowType', WindowType, ...
      |     'bram_latency', bram_latency, ...
      |     'n_inputs', n_inputs, ...
      |     'nput', nput, ...
      |     'fwidth', fwidth);
      settings: AttributesFormatString=PFBSize=8, n_inputs=2, taps=2
  sync_delay : casper_library/Delays/sync_delay  DelayLen=2^(PFBSize-n_inputs)
  dout : Outport
  sync_out : Outport  Port=2
  coeff_out : Outport  Port=3
  taps_out : Outport  Port=4
  wires:
  sync/1 -> pfb_coeff_gen/2(sync)
  din/1 -> pfb_coeff_gen/1(din)
  Mult/1 -> Reinterpret1/1
  pfb_coeff_gen/3(coeff) -> Slice1/1, Slice/1
  pfb_coeff_gen/2(sync_out) -> sync_delay/1
  pfb_coeff_gen/1(dout) -> Reinterpret2/1, delay/1(In1)
  delay/1(Out1) -> dout/1
  sync_delay/1 -> sync_out/1
  Slice1/1 -> coeff_out/1
  Slice/1 -> Reinterpret/1
  Reinterpret/1 -> Mult/2
  Reinterpret1/1 -> taps_out/1
  Reinterpret2/1 -> Mult/1

== system casper_library/PFBs/last_tap ==
  din : Inport  Port=1  LatchInput=off
  sync : Inport  Port=2  LatchInput=off
  coeff : Inport  Port=3  LatchInput=off
  taps : Inport  Port=4  LatchInput=off
  Concat : xbsIndex_r3/Concat  num_inputs=2  explicit_period=off  period=1  dbl_ovrd=off
  Delay : xbsIndex_r3/Delay  latency=mult_latency  reg_retiming=off  explicit_period=off  period=1  en=off  accept_only_valid=off  init_zero=on  dbl_ovrd=off  show_param=off
      settings: xl_area=[0, 0, 0, 0, 0, 0, 0]
  Mult : xbsIndex_r3/Mult  precision=Full  arith_type="Signed  (2's comp)"  n_bits=8  bin_pt=2  quantization=Truncate  overflow=Wrap  latency=mult_latency  explicit_period=off  period=1  en=off  dbl_ovrd=off  show_param=on  mult_type=Parallel  oversample=2  use_embedded=on  pipeline=on  use_rpm=on  placement_style=Rectangular Shape  gen_core=off
      settings: xl_area=[0, 0, 0, 0, 0, 0, 0]
  Mult1 : xbsIndex_r3/Mult  precision=Full  arith_type="Signed  (2's comp)"  n_bits=8  bin_pt=2  quantization=Truncate  overflow=Wrap  latency=mult_latency  explicit_period=off  period=1  en=off  dbl_ovrd=off  show_param=on  mult_type=Parallel  oversample=2  use_embedded=on  pipeline=on  use_rpm=on  placement_style=Rectangular Shape  gen_core=off
      settings: xl_area=[0, 0, 0, 0, 0, 0, 0]
  Reinterpret : xbsIndex_r3/Reinterpret  force_arith_type=on  arith_type="Signed  (2's comp)"  force_bin_pt=on  bin_pt=CoeffBitWidth - 1  force_valid=on
  c_to_ri : casper_library/Misc/c_to_ri  n_bits=BitWidthIn  bin_pt=BitWidthIn-1
      settings: AttributesFormatString=8_7 r/i
  pfb_add_tree : Subsystem  mask(pfb_add_tree){TotalTaps=4, BitWidthIn=8, BitWidthOut=18, CoeffBitWidth=8, add_latency=2, quantization=Truncate}
      mask prompts: TotalTaps "Total Number of Taps:"; BitWidthIn "Input Bitwidth:"; BitWidthOut "Output Bitwidth:"; CoeffBitWidth "Coeff Bitwidth:"; add_latency "Add Latency"; quantization "Quantization Behavior"
      mask init:
      | pfb_add_tree_init(gcb, ...
      |     'TotalTaps', TotalTaps, ...
      |     'BitWidthIn', BitWidthIn, ...
      |     'BitWidthOut', BitWidthOut, ...
      |     'CoeffBitWidth', CoeffBitWidth, ...
      |     'add_latency', add_latency, ...
      |     'quantization', quantization);
      settings: AttributesFormatString=taps=4, add_latency=2
  ri_to_c : Subsystem
  dout : Outport
  sync_out : Outport  Port=2
  wires:
  ri_to_c/1(c) -> Concat/1
  Mult/1 -> ri_to_c/2(im)
  Mult1/1 -> ri_to_c/1(re)
  din/1 -> c_to_ri/1
  c_to_ri/2 -> Mult/1
  c_to_ri/1 -> Mult1/1
  Delay/1 -> pfb_add_tree/2(sync)
  pfb_add_tree/2(sync_out) -> sync_out/1
  pfb_add_tree/1(dout) -> dout/1
  sync/1 -> Delay/1
  taps/1 -> Concat/2
  Concat/1 -> pfb_add_tree/1(din)
  coeff/1 -> Reinterpret/1
  Reinterpret/1 -> Mult1/2, Mult/2
